simulink model "Full_control"  (R2020a)
settings: Solver=VariableStepAuto  StartTime=0.0  StopTime=18  RelTol=1e-3
values from neighbouring files (symbols this model uses):
  Fd = [0 0 9 0 0 0]    [JoinScript.m]    (also in alldata.mat)
  InvMd = inv(Md)    [JoinScript.m]    (also in alldata.mat = [0.01 0 0 0 0 0 0 0.01 0 0 0 0 ... (36 elements, 6x6)])
  K = [C11 C12 C13 0 0 0; C12 C11 C13 0 0 0; C13 C13 C33 0 0 0; 0 0 0 C44 0 0; 0 0 0 0 C44 0; 0 0 0 0 0 C66]    [JoinScript.m]    (also in alldata.mat = [20.1 11.1 12 0 0 0 11.1 20.1 12 0 0 0 ... (36 elements, 6x6; aux_y2.m = Abb.fkine(q))
  Kd = 150*diag([1 1 1 1 1 1])    [JoinScript.m]    (also in alldata.mat = [150 0 0 0 0 0 0 150 0 0 0 0 ... (36 elements, 6x6)]; aux_y.m = 3e2*diag([1 1 1 1 1 1]); aux_y2.m = 3e2*diag([1 1 1 1 1 1]))
  Kp = 200*diag([1 1 1 1 1 1])    [JoinScript.m]    (also in alldata.mat = [200 0 0 0 0 0 0 200 0 0 0 0 ... (36 elements, 6x6)]; aux_y.m = 1e3*diag([1 1 1 1 1 1]); aux_y2.m = 1e3*diag([1 1 1 1 1 1]))
  q0 = [0 0 0 0 0 0 ]    [JoinScript.m]    (also in alldata.mat = [0 0 0 0 0 0]; model_script.m = q; script_trj_q.m = [0 0 0 0 0 0]*pi/180)
  qf = [pi/2 pi/3 pi/12 pi/2 0 pi/2]    [JoinScript.m]    (also in alldata.mat = [1.57079632679 1.0471975512 0.261799387799 1.57079632679 0 1; model_script.m = [pi/6 0 pi/3 pi/4 0 0])
  x0 = dir_kin(qf)    [JoinScript.m]    (also in alldata.mat = [-5.32301496588e-18 0.480120382501 0.16494818601 1.570796326)
settings Model: Creator=doble  LastModifiedBy=doble

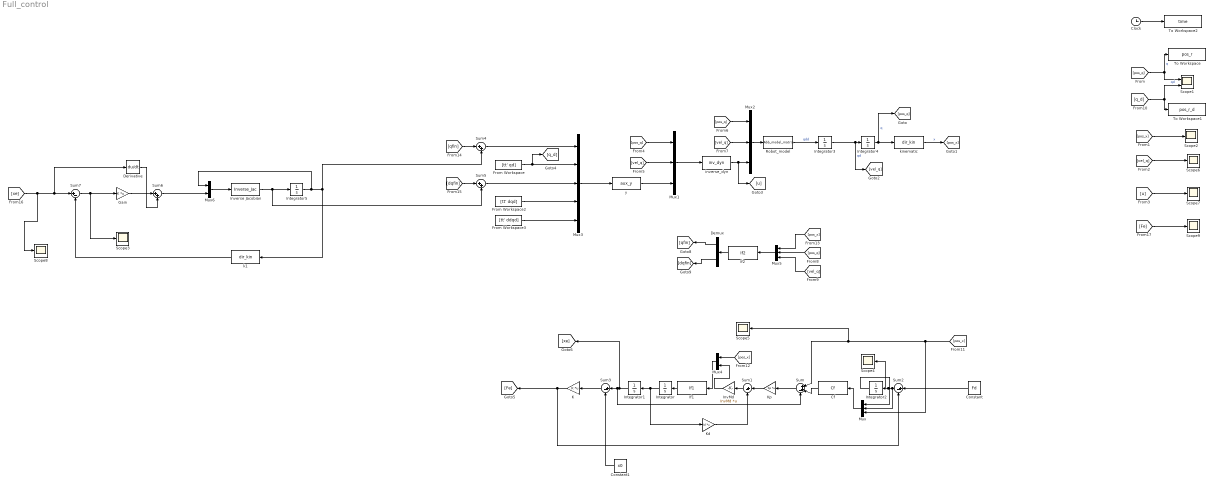
== system Full_control ==
  Cf : MATLABFcn  MATLABFcn=Cf  OutputDimensions=6*1
  Clock : Clock
      settings: Decimation=18
  Constant : Constant  Value=Fd
  Constant1 : Constant  Value=x0
  Demux : Demux  Outputs=[6, 6]
  Derivative : Derivative
  From Workspace : FromWorkspace  VariableName=[tt' qd]
  From Workspace2 : FromWorkspace  VariableName=[tt' dqd]
  From Workspace3 : FromWorkspace  VariableName=[tt' ddqd]
  Gain : Gain  Gain=K  Multiplication=Matrix(K*u)
  If1 : MATLABFcn  MATLABFcn=If1  OutputDimensions=6
  If2 : MATLABFcn  MATLABFcn=If2  OutputDimensions=12
  Integrator : Integrator
  Integrator1 : Integrator  InitialCondition=x0
  Integrator2 : Integrator
  Integrator3 : Integrator
  Integrator4 : Integrator  InitialCondition=q0
  Integrator5 : Integrator  InitialCondition=qf
  InvMd : Gain  Gain=InvMd  Multiplication=Matrix(K*u)
  Inverse Jacobian : MATLABFcn  MATLABFcn=Inverse_Jac  OutputDimensions=6*1
  K : Gain  Gain=K  Multiplication=Matrix(K*u)
  Kd : Gain  Gain=Kd  Multiplication=Matrix(K*u)
  Kp : Gain  Gain=Kp  Multiplication=Matrix(K*u)
  Mux : Mux  Inputs=3
  Mux1 : Mux  Inputs=[6 6 6]
  Mux2 : Mux  Inputs=[6 6 6]
  Mux3 : Mux  Inputs=[6 6 6 6 6]
  Mux4 : Mux  Inputs=2
  Mux5 : Mux  Inputs=3
  Mux6 : Mux  Inputs=[6 6]
  Robot_model : MATLABFcn  MATLABFcn=Abb_model_matrix  OutputDimensions=6
  Scope1 : Scope  NumInputPorts=2
  Scope{2..9} (8 alike) : Scope
  Sum : Sum  Inputs=|++-
  Sum{1..3,7} (4 alike) : Sum  Inputs=|+-
  Sum4 : Sum  Inputs=|++
  Sum5 : Sum  Inputs=|++
  Sum6 : Sum  Inputs=|++
  To Workspace : ToWorkspace  VariableName=pos_r  SampleTime=-1
  To Workspace1 : ToWorkspace  VariableName=pos_r_d  SampleTime=-1
  To Workspace2 : ToWorkspace  VariableName=time  SampleTime=-1
  inverse_dyn : MATLABFcn  MATLABFcn=inv_dyn  OutputDimensions=6
  k1 : MATLABFcn  MATLABFcn=dir_kin
  kinematic : MATLABFcn  MATLABFcn=dir_kin
  y : MATLABFcn  MATLABFcn=aux_y
  wires:
  Sum1/1 -> InvMd/1
  K/1 -> [Fe], Sum2/2
  Sum2/1 -> Integrator2/1, Scope4/1, Mux/2
  Integrator2/1 -> Mux/1
  Mux/1 -> Cf/1
  Constant/1 -> Sum2/1
  Integrator/1 -> Kd/1, Integrator1/1
  Constant1/1 -> Sum3/2
  Kp/1 -> Sum1/1
  Sum/1 -> Kp/1
  Integrator1/1 -> [xe], Sum/3, Sum3/1
  [pos_x] -> Scope5/1, Sum/1, Mux/3
  Kd/1 -> Sum1/2
  Sum3/1 -> K/1
  Cf/1 -> Sum/2
  [pos_x] -> Scope2/1
  From Workspace3/1 -> Mux3/5
  Mux1/1 -> inverse_dyn/1
  y/1 -> Mux1/3
  [vel_q] -> Scope6/1
  Mux3/1 -> y/1
  [u] -> Scope7/1
  [vel_q] -> Mux2/2
  [pos_q] -> Mux1/1
  Clock/1 -> To Workspace2/1
  From Workspace2/1 -> Mux3/4
  From Workspace/1 -> Mux3/2, [q_d]
  Integrator4/1 -> [pos_q], kinematic/1  "q"
  Sum5/1 -> Mux3/3
  Sum4/1 -> Mux3/1
  kinematic/1 -> [pos_x]  "x"
  [vel_q] -> Mux1/2
  [pos_q] -> To Workspace/1, Scope1/1  "q"
  [q_d] -> To Workspace1/1, Scope1/2  "qd"
  [pos_q] -> Mux2/1
  Mux2/1 -> Robot_model/1
  inverse_dyn/1 -> Mux2/3, [u]
  Integrator3/1 -> [vel_q], Integrator4/1  "qd"
  Robot_model/1 -> Integrator3/1  "qdd"
  If1/1 -> Integrator/1
  InvMd/1 -> Mux4/2
  [pos_x] -> Mux4/1
  Mux4/1 -> If1/1
  Mux5/1 -> If2/1
  If2/1 -> Demux/1
  [vel_q] -> Mux5/3
  [pos_q] -> Mux5/2
  [pos_x] -> Mux5/1
  Demux/1 -> [qfin]
  Demux/2 -> [dqfin]
  [qfin] -> Sum4/1
  [dqfin] -> Sum5/1
  Derivative/1 -> Sum6/2
  k1/1 -> Sum7/2
  Integrator5/1 -> Mux6/1, Sum4/2, k1/1
  Sum7/1 -> Scope3/1, Gain/1
  Gain/1 -> Sum6/1
  Sum6/1 -> Mux6/2
  [xe] -> Derivative/1, Sum7/1, Scope8/1
  Inverse Jacobian/1 -> Sum5/2, Integrator5/1
  Mux6/1 -> Inverse Jacobian/1
  [Fe] -> Scope9/1
